simulink model "simulink_Controler_Xi"  (R2014a)
settings: Solver=ode45  StartTime=0.0  StopTime=2  RelTol=1e-3
values from neighbouring files (symbols this model uses):
  A = [0 1 0 0 ... (first row only)    [ME531_Project_Xi.m]
  B = [0 0 ... (first row only)    [ME531_Project_Xi.m]
  C = eye(4)    [ME531_Project_Xi.m]
  D = [0 0 ;0 0;0 0;0 0]    [ME531_Project_Xi.m]
  x0 = [d0; 0; th0; 0]    [ME531_Project_Xi.m]
  xTarget = [d0;  0; atan(aSys/g); 0]    [ME531_Project_Xi.m]
undefined symbols (not defined in the file or in its folder): k
settings Model: Creator=Fisher  LastModifiedBy=Fisher

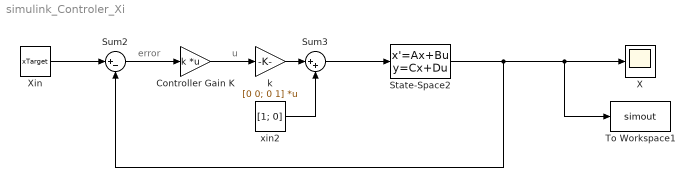
== system simulink_Controler_Xi ==
  note: u
  note: error
  Controller Gain K : Gain  Gain=k  Multiplication=Matrix(K*u)
  State-Space2 : StateSpace  A=A  B=B  C=C  D=D  X0=x0
  Sum2 : Sum  Inputs=|+-
  Sum3 : Sum  Inputs=|++
  To Workspace1 : ToWorkspace  VariableName=simout  SaveFormat=Timeseries  SampleTime=-1
  X : Scope
      settings: TimeRange=10  YMin=-2  YMax=8
  Xin : Constant  Value=xTarget
  k : Gain  Gain=[0 0; 0 1]  Multiplication=Matrix(K*u)
  xin2 : Constant  Value=[1; 0]
  wires:
  State-Space2/1 -> To Workspace1/1, X/1, Sum2/2
  Xin/1 -> Sum2/1
  Sum2/1 -> Controller Gain K/1
  xin2/1 -> Sum3/2
  k/1 -> Sum3/1
  Controller Gain K/1 -> k/1
  Sum3/1 -> State-Space2/1
